simulink subsystem "No_Chain_Drive"  (R2025b)
settings: Solver=VariableStepAuto  StartTime=0.0  StopTime=10.0  RelTol=1e-3
settings Model: Creator=The MathWorks, Inc.  LastModifiedBy=The MathWorks, Inc.
settings RTWCC: GPUComputeCapability=3.5

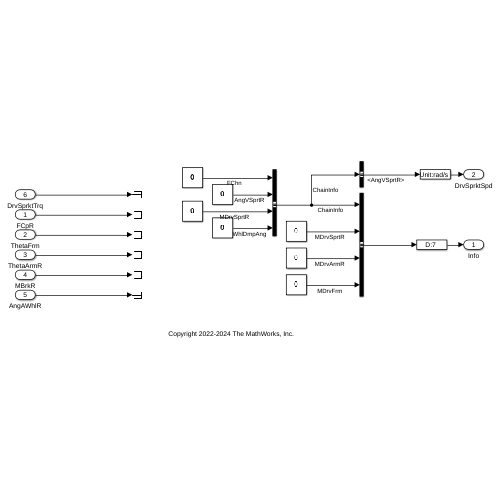
[thumbnail: Simulink's stored preview of the top-level diagram]
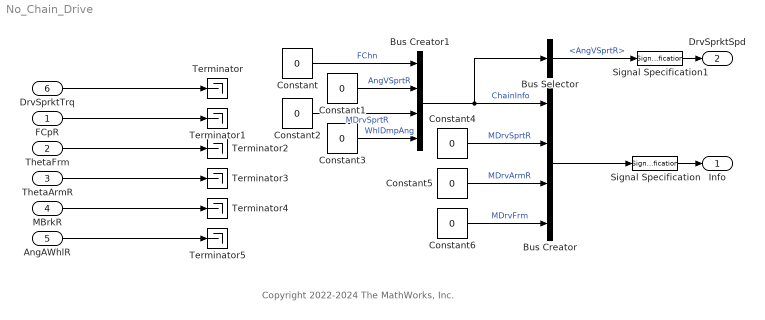
== system No_Chain_Drive ==
  note: Copyright 2022-2024 The MathWorks, Inc.
  FCpR : Inport
  ThetaFrm : Inport  Port=2
  ThetaArmR : Inport  Port=3
  MBrkR : Inport  Port=4
  AngAWhlR : Inport  Port=5
  DrvSprktTrq : Inport  Port=6
  Bus Creator : BusCreator  Inputs=4
  Bus Creator1 : BusCreator  Inputs=4
  Bus Selector : BusSelector  OutputSignals=AngVSprtR
  Constant{,1..6} (7 alike) : Constant  Value=0
  Signal Specification : SignalSpecification  Dimensions=7
  Signal Specification1 : SignalSpecification  Unit=rad/s
  Terminator{,1..5} (6 alike) : Terminator
  Info : Outport
  DrvSprktSpd : Outport  Port=2
  wires:
  Constant6/1 -> Bus Creator/4  "MDrvFrm"
  Bus Creator/1 -> Signal Specification/1
  Constant5/1 -> Bus Creator/3  "MDrvArmR"
  Constant4/1 -> Bus Creator/2  "MDrvSprtR"
  FCpR/1 -> Terminator1/1
  ThetaFrm/1 -> Terminator2/1
  DrvSprktTrq/1 -> Terminator/1
  MBrkR/1 -> Terminator4/1
  Signal Specification/1 -> Info/1
  AngAWhlR/1 -> Terminator5/1
  ThetaArmR/1 -> Terminator3/1
  Constant/1 -> Bus Creator1/1  "FChn"
  Constant1/1 -> Bus Creator1/2  "AngVSprtR"
  Constant2/1 -> Bus Creator1/3  "MDrvSprtR"
  Constant3/1 -> Bus Creator1/4  "WhlDmpAng"
  Bus Creator1/1 -> Bus Creator/1, Bus Selector/1  "ChainInfo"
  Bus Selector/1 -> Signal Specification1/1  "<AngVSprtR>"
  Signal Specification1/1 -> DrvSprktSpd/1
